simulink model "Derrame_tk"  (R2020b)
settings: Solver=VariableStepAuto  StartTime=0.0  StopTime=10  RelTol=1e-3
settings Model: Creator=retou  LastModifiedBy=retou

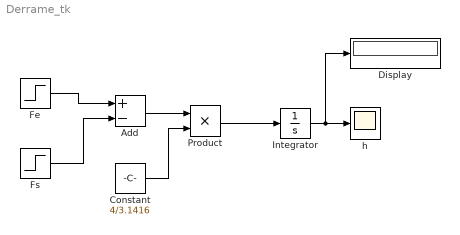
== system Derrame_tk ==
  Add : Sum  Inputs=+-
  Constant : Constant  Value=4/3.1416
  Display : Display
  Fe : Step  Time=0  Before=0.1  After=0.1  SampleTime=0
  Fs : Step  Time=0  Before=0.1  After=0  SampleTime=0
  Integrator : Integrator  InitialCondition=1
  Product : Product
  h : Scope
  wires:
  Fe/1 -> Add/1
  Fs/1 -> Add/2
  Add/1 -> Product/1
  Constant/1 -> Product/2
  Product/1 -> Integrator/1
  Integrator/1 -> Display/1, h/1
